simulink model "uncontrolled_group24"  (R2023b)
settings: Solver=ode5  StartTime=0.0  StopTime=333  FixedStep=0.1  RelTol=1e-3
values from neighbouring files (symbols this model uses):
  a = 6939    [Air_Drag_script.m]    (also in main.m = 6939.063; main_group24.m = 6939.063)
  A0 = eye(3)    [Air_Drag_script.m]    (also in main_group24.m)
  ARW = 0.15    [main_group24.m]
  c = 2.99792*10^8    (= 299792000)    [main.m]    (also in main_group24.m)
  e = 0    [Air_Drag_script.m]    (also in main.m = 0.001304; main_group24.m)
  G = [gn, gm, gvali, gsvi]    [main.m]    (also in main_group24.m)
  GyroSampleRate = 10    [main_group24.m]
  H = [hn, hm, hvali, hsvi]    [main.m]    (also in main_group24.m)
  i = deg2rad(97.5307)    [Air_Drag_script.m]    (also in main.m; main_group24.m)
  I_tot = [Ix 0 0; 0 Iy 0; 0 0 Iz]    [data_mass.m]    (also in main_group24.m)
  invI_tot = inv(I_tot)    [data_mass.m]    (also in main_group24.m)
  Ix = J(1,1)    [Air_Drag_script.m]    (also in data_mass.m = 0.0755003333333; main.m = 0.057749855; main_group24.m = 0.0755003333333)
  Iy = J(2,2)    [Air_Drag_script.m]    (also in data_mass.m = 0.0755003333333; main.m = 0.04143542; main_group24.m = 0.0755003333333)
  Iz = J(3,3)    [Air_Drag_script.m]    (also in data_mass.m = 0.055; main.m = 0.024624309; main_group24.m = 0.055)
  m = [0.1; 0.1; 0.1]    [main.m]    (also in main_group24.m)
  MB = [4; 0.1; 0.1; 0.3]    [main.m]    (also in main_group24.m)
  MMnoise = 15e-9*[1; 1; 1]    [main_group24.m]
  MMSampleRate = 1    [main_group24.m]
  mu = 3.98600433e+5    (= 398600.433)    [main.m]    (also in main_group24.m)
  n = 0.0011    [Air_Drag_script.m]    (also in main.m = sqrt(mu/a^3); main_group24.m = sqrt(mu/a^3))
  q0 = [ 1 1 1 1 ]'    [Air_Drag_script.m]    (also in main_group24.m = [0 0 0 1]')
  R_e = 6378    [main.m]    (also in main_group24.m)
  rho_air = 1.65e-13    [Air_Drag_script.m]
  rho_d_MB = 0.1    [main.m]    (also in main_group24.m)
  rho_d_SP = 0.1    [main.m]    (also in main_group24.m)
  rho_s_MB = 0.5    [main.m]    (also in main_group24.m)
  rho_s_SP = 0.1    [main.m]    (also in main_group24.m)
  RRW = 0.3    [main_group24.m]
  SP = [1; 0.3; 0.1; 0.01]    [main.m]    (also in main_group24.m = [0.25; 0.1; 0.3; 0.01])
  w0 = [0 0 0]'    [Air_Drag_script.m]    (also in main.m = [wx0; wy0; wz0]; main_group24.m = [wx0; wy0; wz0])
undefined symbols (not defined in the file or in its folder): Cd, H_0, n_E, P, pan1, pan2, rho_d_body, rho_d_sp, rho_s_body, rho_s_sp, s1, s2, s3, s4, s5, s6, v_rel
libraries: vrlib x40, simulink_extras x13, matrix_library x8, sharedutil x3, simulink x1
(part 2 of 4)

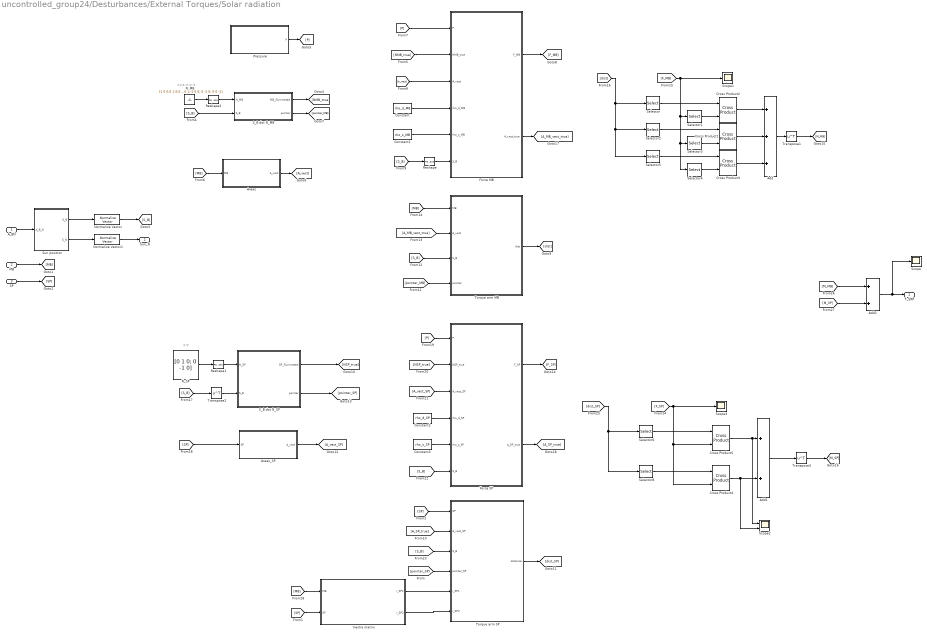
== system uncontrolled_group24/Desturbances/External Torques/Solar radiation ==
  note: x,y,z,-x,-y,-z
  note: y,-y
  A_BN : Inport
  MB : Inport  Port=2
  SP : Inport  Port=3
  Add : Sum  Inputs=3
  Add1 : Sum
  Add2 : Sum
  Areas : Subsystem
  Areas_SP : Subsystem
  Constant : Constant  Value=rho_d_MB
  Constant1 : Constant  Value=rho_s_MB
  Constant2 : Constant  Value=rho_d_SP
  Constant3 : Constant  Value=rho_s_SP
  Cross Product{1..5} (5 alike) : matrix_library/Cross Product
  Force MB : Subsystem
  Force SP : Subsystem
  Inertia matrix : Subsystem
  N_MB : Constant  Value=[1 0 0;0 1 0;0 0 1;-1 0 0; 0 -1 0; 0 0 -1]  VectorParams1D=off
  N_SP : Constant  Value=[0 1 0; 0 -1 0]  VectorParams1D=off
  Normalize Vector : vrlib/Utilities/Normalize Vector  maxzero=0
  Normalize Vector1 : vrlib/Utilities/Normalize Vector  maxzero=0
  Pressure : Subsystem
  Reshape : Reshape  OutputDimensionality=Column vector (2-D)
  Reshape1 : Reshape  OutputDimensionality=Customize  OutputDimensions=[2,3]
  Reshape2 : Reshape  OutputDimensionality=Customize  OutputDimensions=[6,3]
  S_B dot N_MB : Subsystem
  S_B dot N_SP : Subsystem
  Scope : Scope
  Scope1 : Scope
  Scope2 : Scope  NumInputPorts=2
  Scope3 : Scope
  Selector : Selector  NumberOfDimensions=2  InputPortWidth=3  IndexOptions=Index vector (dialog),Index vector (dialog)  Indices=1,[1 2 3]  OutputSizes=1,1
  Selector1 : Selector  NumberOfDimensions=2  InputPortWidth=3  IndexOptions=Index vector (dialog),Index vector (dialog)  Indices=1,[1 2 3]  OutputSizes=1,1
  Selector2 : Selector  NumberOfDimensions=2  InputPortWidth=3  IndexOptions=Index vector (dialog),Index vector (dialog)  Indices=2,[1 2 3]  OutputSizes=1,1
  Selector3 : Selector  NumberOfDimensions=2  InputPortWidth=3  IndexOptions=Index vector (dialog),Index vector (dialog)  Indices=2,[1 2 3]  OutputSizes=1,1
  Selector4 : Selector  NumberOfDimensions=2  InputPortWidth=3  IndexOptions=Index vector (dialog),Index vector (dialog)  Indices=3,[1 2 3]  OutputSizes=1,1
  Selector5 : Selector  NumberOfDimensions=2  InputPortWidth=3  IndexOptions=Index vector (dialog),Index vector (dialog)  Indices=3,[1 2 3]  OutputSizes=1,1
  Selector6 : Selector  NumberOfDimensions=2  InputPortWidth=3  IndexOptions=Index vector (dialog),Index vector (dialog)  Indices=1,[1 2 3]  OutputSizes=1,1
  Selector8 : Selector  NumberOfDimensions=2  InputPortWidth=3  IndexOptions=Index vector (dialog),Index vector (dialog)  Indices=2,[1 2 3]  OutputSizes=1,1
  Sun position : Subsystem
  Torque arm MB : Subsystem
  Torque arm SP : Subsystem
  Transpose1 : Math  Operator=transpose
  Transpose2 : Math  Operator=transpose
  Transpose3 : Math  Operator=transpose
  T_SRP : Outport
  Sun_N : Outport  Port=2
  wires:
  Sun position/1(S_B) -> Normalize Vector/1
  MB/1 -> [MB]
  N_MB/1 -> Reshape2/1
  [NMB_true] -> Force MB/2(NMB_true)
  S_B dot N_MB/1(MB_illuminated) -> [NMB_true]
  [MB] -> Areas/1(MB)
  [S_B] -> S_B dot N_MB/2(S_B)
  [P] -> Force MB/1(P)
  Areas/1(A_vect) -> [A_vect]
  Transpose1/1 -> [M_MB]
  Areas_SP/1(A_vect) -> [A_vect_SP]
  Reshape1/1 -> S_B dot N_SP/1(N_SP)
  Transpose3/1 -> [M_SP]
  Selector2/1 -> Cross Product1/1
  [MB] -> Torque arm MB/1(MB)
  Constant3/1 -> Force SP/5(rho_s_SP)
  [F_SP] -> Cross Product5/2, Cross Product4/2, Scope3/1
  [M_MB] -> Add2/1
  [dist_SP] -> Selector6/1, Selector8/1
  [pointer_SP] -> Torque arm SP/4(pointer_SP)
  Cross Product4/1 -> Scope2/2, Add1/2
  [F_MB] -> Scope1/1, Selector4/1, Selector3/1, Selector1/1
  A_BN/1 -> Sun position/1(A_B_N)
  Add1/1 -> Transpose3/1
  Transpose2/1 -> S_B dot N_SP/2(S_B)
  [SP] -> Areas_SP/1(SP)
  [A_SP_true] -> Torque arm SP/2(A_vect_SP)
  Add/1 -> Transpose1/1
  Torque arm SP/1(distance) -> [dist_SP]
  Reshape2/1 -> S_B dot N_MB/1(N_MB)
  Torque arm MB/1(dist) -> [dist]
  S_B dot N_SP/2(pointer) -> [pointer_SP]
  Force MB/1(F_MB) -> [F_MB]
  Selector/1 -> Cross Product2/1
  [S_B] -> Reshape/1
  [P] -> Force SP/1(P)
  [A_vect] -> Force MB/3(A_vect)
  Selector1/1 -> Cross Product2/2
  Constant1/1 -> Force MB/5(rho_s_MB)
  [A_MB_vect_true] -> Torque arm MB/2(A_vect)
  Pressure/1(P) -> [P]
  Normalize Vector/1 -> [S_B]
  Constant2/1 -> Force SP/4(rho_d_SP)
  Constant/1 -> Force MB/4(rho_d_MB)
  Selector8/1 -> Cross Product4/1
  [dist] -> Selector2/1, Selector5/1, Selector/1
  [NSP_true] -> Force SP/2(NSP_true)
  N_SP/1 -> Reshape1/1
  [S_B] -> Torque arm MB/3(S_B)
  Force SP/2(A_SP_true) -> [A_SP_true]
  [S_B] -> Torque arm SP/3(S_B)
  SP/1 -> [SP]
  Selector4/1 -> Cross Product3/2
  S_B dot N_MB/2(pointer) -> [pointer_MB]
  Force MB/2(A_vect_true) -> [A_MB_vect_true]
  [pointer_MB] -> Torque arm MB/4(pointer)
  Add2/1 -> Scope/1, T_SRP/1
  Selector3/1 -> Cross Product1/2
  [S_B] -> Force SP/6(S_B)
  [S_B] -> Transpose2/1
  Cross Product5/1 -> Scope2/1, Add1/1
  [A_vect_SP] -> Force SP/3(A_vect_SP)
  Reshape/1 -> Force MB/6(S_B)
  Cross Product2/1 -> Add/1
  Force SP/1(F_SP) -> [F_SP]
  S_B dot N_SP/1(SP_illuminated) -> [NSP_true]
  Selector6/1 -> Cross Product5/1
  Selector5/1 -> Cross Product3/1
  Cross Product1/1 -> Add/2
  [M_SP] -> Add2/2
  [SP] -> Torque arm SP/1(SP)
  Cross Product3/1 -> Add/3
  [SP] -> Inertia matrix/2(SP)
  [MB] -> Inertia matrix/1(MB)
  Inertia matrix/1(r_SP1) -> Torque arm SP/5(r_SP1)
  Inertia matrix/2(r_SP2) -> Torque arm SP/6(r_SP2)
  Sun position/2(S_N) -> Normalize Vector1/1
  Normalize Vector1/1 -> Sun_N/1

== system uncontrolled_group24/Desturbances/Orbital Mechanics/Sat Position magnitude ==
  note: 1+e cos(theta)
  note: a(1-e^2)
  note: Denominator
  note: Numerator
  theta : Inport
  Constant : Constant  Value=a
  Constant1 : Constant
  Constant3 : Constant  Value=e
  Constant4 : Constant
  Constant5 : Constant  Value=e
  Cos : Trigonometry  Operator=cos
  Divide : Product  Inputs=*/
  Product : Product
  Product1 : Product
  Square1 : Math  Operator=square
  Sum : Sum
  Sum1 : Sum  Inputs=+-
  r : Outport
  wires:
  Product1/1 -> Sum/1
  Sum1/1 -> Product/2
  Constant1/1 -> Sum1/1
  Sum/1 -> Divide/2
  Square1/1 -> Sum1/2
  Constant3/1 -> Product1/2
  Constant4/1 -> Sum/2
  Constant/1 -> Product/1
  Constant5/1 -> Square1/1
  Cos/1 -> Product1/1
  Product/1 -> Divide/1
  theta/1 -> Cos/1
  Divide/1 -> r/1

== system uncontrolled_group24/Desturbances/Orbital Mechanics/Sat True Anomaly ==
  note: (1-e^2)^3/2
  note: n ( 1+e cos(theta))^2
  note: Denominator
  note: Numerator
  Constant : Constant  Value=n
  Constant1 : Constant
  Constant2 : Constant  Value=e
  Constant3 : Constant
  Constant4 : Constant  Value=e
  Constant5 : Constant  Value=3/2
  Cos : Trigonometry  Operator=cos
  Divide : Product  Inputs=*/
  Integrator : Integrator
  Power : Math  Operator=pow
  Product : Product
  Product1 : Product
  Square : Math  Operator=square
  Square1 : Math  Operator=square
  Sum : Sum
  Sum1 : Sum  Inputs=|+-
  theta : Outport
  wires:
  Sum/1 -> Square/1
  Integrator/1 -> theta/1, Cos/1  "theta"
  Square/1 -> Product1/2
  Constant5/1 -> Power/2
  Constant3/1 -> Sum1/1
  Product1/1 -> Divide/1
  Constant/1 -> Product1/1
  Divide/1 -> Integrator/1  "theta_dot"
  Square1/1 -> Sum1/2
  Product/1 -> Sum/2
  Power/1 -> Divide/2
  Constant1/1 -> Sum/1
  Constant2/1 -> Product/1
  Constant4/1 -> Square1/1
  Cos/1 -> Product/2
  Sum1/1 -> Power/1

== system uncontrolled_group24/Desturbances/Orbital Mechanics/Sat position vector in inertial frame ==
  note: r_N = r [cos(theta)
      | 		sin(theta)cos(i)
      | 		sin(theta)sin(i)]
  r : Inport
  theta : Inport  Port=2
  Cos : Trigonometry  Operator=cos
  Cos1 : Trigonometry  Operator=cos
  Orbit Inclination : Constant  Value=i
  Product : Product
  Product1 : Product
  Product2 : Product
  Sin : Trigonometry
  Sin1 : Trigonometry
  Vector Concatenate : Concatenate  NumInputs=3  Mode=Multidimensional array
  r_N : Outport
  wires:
  Sin/1 -> Product1/1, Product/1
  Product/1 -> Vector Concatenate/2
  Sin1/1 -> Product1/2
  r/1 -> Product2/1
  Orbit Inclination/1 -> Sin1/1, Cos1/1
  Vector Concatenate/1 -> Product2/2
  theta/1 -> Cos/1, Sin/1
  Cos/1 -> Vector Concatenate/1
  Cos1/1 -> Product/2
  Product1/1 -> Vector Concatenate/3
  Product2/1 -> r_N/1

== system uncontrolled_group24/Desturbances/Relative Attitude/A_BL ==
  A_BN : Inport
  A_LN : Inport  Port=2
  Matrix Multiply : Product  Multiplication=Matrix(*)
  To Workspace : ToWorkspace  VariableName=A_BL  SampleTime=-1
  Transpose1 : matrix_library/Transpose
  A_BL : Outport
  wires:
  A_BN/1 -> Matrix Multiply/1
  A_LN/1 -> Transpose1/1
  Transpose1/1 -> Matrix Multiply/2
  Matrix Multiply/1 -> A_BL/1, To Workspace/1

== system uncontrolled_group24/Desturbances/Relative Attitude/A_LN ==
  theta : Inport
  Constant : Constant  Value=0
  Constant1 : Constant  Value=[0; 0; 1]
  Constant2 : Constant  Value=[1 0 0; 0 cos(i) sin(i); 0 -sin(i) cos(i)]
  Cos : Trigonometry  Operator=cos
  Gain : Gain  Gain=[1; -1; 1]
  Matrix Concatenate : Concatenate  NumInputs=3  Mode=Multidimensional array  ConcatenateDimension=2
  Product : Product  Multiplication=Matrix(*)
  Selector : Selector  InputPortWidth=3  IndexOptions=Index vector (dialog)  Indices=[3 2 1]  OutputSizes=1
  Selector1 : Selector  InputPortWidth=3  IndexOptions=Index vector (dialog)  Indices=[2 3 1]  OutputSizes=1
  Sin : Trigonometry
  To Workspace : ToWorkspace  VariableName=A_LN  SampleTime=-1
  Vector Concatenate : Concatenate  NumInputs=3
  A_LN : Outport
  wires:
  Matrix Concatenate/1 -> Product/1
  theta/1 -> Sin/1, Cos/1
  Gain/1 -> Matrix Concatenate/1
  Vector Concatenate/1 -> Selector1/1, Selector/1
  Sin/1 -> Vector Concatenate/3
  Selector/1 -> Matrix Concatenate/2
  Selector1/1 -> Gain/1
  Product/1 -> A_LN/1, To Workspace/1
  Constant1/1 -> Matrix Concatenate/3
  Cos/1 -> Vector Concatenate/2
  Constant/1 -> Vector Concatenate/1
  Constant2/1 -> Product/2

== system uncontrolled_group24/Sensors/Magnetometer/Subsystem ==
  Constant : Constant
  Display : Display
  Gain : Gain  Gain=[1; -1; 1]
  Gain1 : Gain  Gain=[1; 1; -1]
  Gain2 : Gain  Gain=[-1; 1; 1]
  Matrix Concatenate : Concatenate  NumInputs=3  Mode=Multidimensional array  ConcatenateDimension=2
  Random Number : RandomNumber  Variance=deg2rad(0.1)^2  Seed=5  SampleTime=1/MMSampleRate
  Random Number1 : RandomNumber  Variance=deg2rad(0.1)^2  Seed=6  SampleTime=1/MMSampleRate
  Random Number2 : RandomNumber  Variance=deg2rad(0.1)^2  Seed=7  SampleTime=1/MMSampleRate
  Selector : Selector  InputPortWidth=4  IndexOptions=Index vector (dialog)  Indices=[1 4 3]  OutputSizes=1
  Selector1 : Selector  InputPortWidth=4  IndexOptions=Index vector (dialog)  Indices=[4 1 2]  OutputSizes=1
  Selector2 : Selector  InputPortWidth=4  IndexOptions=Index vector (dialog)  Indices=[3 2 1]  OutputSizes=1
  Vector Concatenate : Concatenate  NumInputs=4
  A_epsMM : Outport
  wires:
  Selector2/1 -> Gain2/1
  Selector/1 -> Gain/1
  Gain/1 -> Matrix Concatenate/1
  Random Number/1 -> Vector Concatenate/2
  Matrix Concatenate/1 -> Display/1, A_epsMM/1
  Selector1/1 -> Gain1/1
  Vector Concatenate/1 -> Selector2/1, Selector/1, Selector1/1
  Gain2/1 -> Matrix Concatenate/3
  Constant/1 -> Vector Concatenate/1
  Gain1/1 -> Matrix Concatenate/2
  Random Number2/1 -> Vector Concatenate/4
  Random Number1/1 -> Vector Concatenate/3

== system uncontrolled_group24/Sensors/Sun Sensor/Subsystem ==
  note: A31
  note: A33
  note: A32
  note: A23
  note: A22
  note: A21
  note: A13
  note: A12
  note: A11
  Cos : Trigonometry  Operator=cos
  Cos1 : Trigonometry  Operator=cos
  Cos2 : Trigonometry  Operator=cos
  Create 3x3 Matrix : sharedutil/Create 3x3 Matrix  aMode=aMode
  Gain1 : Gain  Gain=-1
  Gain3 : Gain  Gain=-1
  Gain4 : Gain
  Product{,1,3,5..6,8,10..11} (8 alike) : Product
  Product{2,4,7,9} (4 alike) : Product  Inputs=3
  Sin : Trigonometry
  Sin1 : Trigonometry
  Sin2 : Trigonometry
  Sum : Sum
  Sum1 : Sum  Inputs=-+
  Sum2 : Sum  Inputs=-+
  Sum3 : Sum
  phi : RandomNumber  Variance=(1/8*pi/180)^2  Seed=2  SampleTime=0.2
  psi : RandomNumber  Variance=(1/8*pi/180)^2  SampleTime=0.2
  th : RandomNumber  Variance=(1/8*pi/180)^2  Seed=1  SampleTime=0.2
  A_eps : Outport
  wires:
  psi/1 -> Cos/1, Sin/1
  th/1 -> Sin1/1, Cos1/1
  phi/1 -> Sin2/1, Cos2/1
  Product2/1 -> Sum/1
  Product1/1 -> Sum/2
  Product3/1 -> Sum1/2
  Product4/1 -> Sum1/1
  Product7/1 -> Sum2/1
  Product6/1 -> Sum2/2
  Product9/1 -> Sum3/1
  Product8/1 -> Sum3/2
  Gain4/1 -> Create 3x3 Matrix/7  "A31"
  Product/1 -> Create 3x3 Matrix/1  "A11"
  Sum/1 -> Create 3x3 Matrix/2  "A12"
  Sum1/1 -> Create 3x3 Matrix/3  "A13"
  Product5/1 -> Gain1/1
  Sum2/1 -> Create 3x3 Matrix/5  "A22"
  Sum3/1 -> Create 3x3 Matrix/6  "A23"
  Product10/1 -> Gain3/1
  Product11/1 -> Create 3x3 Matrix/9  "A33"
  Gain1/1 -> Create 3x3 Matrix/4  "A21"
  Gain3/1 -> Create 3x3 Matrix/8  "A32"
  Cos/1 -> Product8/1, Product6/1, Product4/1, Product2/1, Product/1  "cos(psi)"
  Cos1/1 -> Product/2, Product11/1, Product10/1, Product5/2  "cos(th)"
  Sin1/1 -> Gain4/1, Product9/2, Product7/2, Product2/2, Product4/2  "sin(th)"
  Sin2/1 -> Product7/3, Product3/2, Product2/3, Product8/2, Product10/2  "sin(phi)"
  Sin/1 -> Product3/1, Product5/1, Product7/1, Product9/1, Product1/1  "sin(psi)"
  Cos2/1 -> Product6/2, Product4/3, Product1/2, Product9/3, Product11/2  "cos(phi)"
  Create 3x3 Matrix/1 -> A_eps/1  "A_eps"

== system uncontrolled_group24/errormeasure/IJK_error/I_Error ==
  A_BN_estimated : Inport
  I : Inport  Port=2
  A_B_N_ea : Inport  Port=3
  Acos : Trigonometry  Operator=acos
  Dot Product : DotProduct  OutDataTypeStr=Inherit: Inherit via internal rule
  MatrixMultiply : Product  Multiplication=Matrix(*)
  MatrixMultiply1 : Product  Multiplication=Matrix(*)
  Normalize Vector : vrlib/Utilities/Normalize Vector  maxzero=0
  Normalize Vector1 : vrlib/Utilities/Normalize Vector  maxzero=0
  Radians to Degrees : simulink_extras/Transformations/Radians to Degrees
  Degrees out : Outport
  wires:
  MatrixMultiply1/1 -> Normalize Vector/1
  Dot Product/1 -> Acos/1
  I/1 -> MatrixMultiply1/2, MatrixMultiply/2
  Normalize Vector1/1 -> Dot Product/2
  Normalize Vector/1 -> Dot Product/1
  Acos/1 -> Radians to Degrees/1  "Theta_err"
  A_BN_estimated/1 -> MatrixMultiply1/1
  MatrixMultiply/1 -> Normalize Vector1/1
  A_B_N_ea/1 -> MatrixMultiply/1
  Radians to Degrees/1 -> Degrees out/1

== system uncontrolled_group24/errormeasure/IJK_error/J_Error ==
  A_BN_estimated : Inport
  J : Inport  Port=2
  A_B_N_ea : Inport  Port=3
  Acos : Trigonometry  Operator=acos
  Dot Product : DotProduct  OutDataTypeStr=Inherit: Inherit via internal rule
  MatrixMultiply : Product  Multiplication=Matrix(*)
  MatrixMultiply1 : Product  Multiplication=Matrix(*)
  Normalize Vector : vrlib/Utilities/Normalize Vector  maxzero=0
  Normalize Vector1 : vrlib/Utilities/Normalize Vector  maxzero=0
  Radians to Degrees : simulink_extras/Transformations/Radians to Degrees
  Degrees out : Outport
  wires:
  MatrixMultiply1/1 -> Normalize Vector/1
  Dot Product/1 -> Acos/1
  J/1 -> MatrixMultiply1/2, MatrixMultiply/2
  Normalize Vector1/1 -> Dot Product/2
  Normalize Vector/1 -> Dot Product/1
  Acos/1 -> Radians to Degrees/1  "Theta_err"
  A_BN_estimated/1 -> MatrixMultiply1/1
  MatrixMultiply/1 -> Normalize Vector1/1
  A_B_N_ea/1 -> MatrixMultiply/1
  Radians to Degrees/1 -> Degrees out/1

== system uncontrolled_group24/errormeasure/IJK_error/K_Error ==
  A_BN_estimated : Inport
  K : Inport  Port=2
  A_B_N_ea : Inport  Port=3
  Acos : Trigonometry  Operator=acos
  Dot Product : DotProduct  OutDataTypeStr=Inherit: Inherit via internal rule
  MatrixMultiply : Product  Multiplication=Matrix(*)
  MatrixMultiply1 : Product  Multiplication=Matrix(*)
  Normalize Vector : vrlib/Utilities/Normalize Vector  maxzero=0
  Normalize Vector1 : vrlib/Utilities/Normalize Vector  maxzero=0
  Radians to Degrees : simulink_extras/Transformations/Radians to Degrees
  Degrees out : Outport
  wires:
  MatrixMultiply1/1 -> Normalize Vector/1
  Dot Product/1 -> Acos/1
  K/1 -> MatrixMultiply1/2, MatrixMultiply/2
  Normalize Vector1/1 -> Dot Product/2
  Normalize Vector/1 -> Dot Product/1
  Acos/1 -> Radians to Degrees/1  "Theta_err"
  A_BN_estimated/1 -> MatrixMultiply1/1
  MatrixMultiply/1 -> Normalize Vector1/1
  A_B_N_ea/1 -> MatrixMultiply/1
  Radians to Degrees/1 -> Degrees out/1

== system uncontrolled_group24/Desturbances/External Torques/M_GG/GG Torque1 ==
  c1 : Inport
  c2 : Inport  Port=2
  c3 : Inport  Port=3
  r : Inport  Port=4
  Constant5 : Constant  Value=3
  Constant6 : Constant  Value=3*mu
  Divide3 : Product  Inputs=*/
  Gain1 : Gain  Gain=Iz-Iy
  Gain2 : Gain  Gain=Ix-Iz
  Gain3 : Gain  Gain=Iy-Ix
  Mux1 : Mux  Inputs=3
  Pow1 : Math  Operator=pow  RndMeth=Zero
  Product{1..2,6..9} (6 alike) : Product
  M_GG : Outport
  wires:
  Gain1/1 -> Mux1/1
  Product7/1 -> Gain1/1
  Gain3/1 -> Mux1/3
  Product2/1 -> Product8/1
  r/1 -> Pow1/1
  Product6/1 -> Product9/1
  Product1/1 -> Product7/1
  Constant6/1 -> Divide3/1
  Product8/1 -> Gain2/1
  Pow1/1 -> Divide3/2
  c2/1 -> Product6/2, Product1/1
  Mux1/1 -> M_GG/1
  Product9/1 -> Gain3/1
  Constant5/1 -> Pow1/2
  Gain2/1 -> Mux1/2
  c3/1 -> Product1/2, Product2/2
  c1/1 -> Product6/1, Product2/1
  Divide3/1 -> Product7/2, Product8/2, Product9/2

== system uncontrolled_group24/Desturbances/External Torques/M_GG/c1, c2, c3 ==
  A_BL : Inport
  Constant1 : Constant  Value=[1; 0; 0]
  Demux : Demux  Outputs=3
  Product1 : Product  Multiplication=Matrix(*)
  c1 : Outport
  c2 : Outport  Port=2
  c3 : Outport  Port=3
  wires:
  Demux/2 -> c2/1
  Product1/1 -> Demux/1
  Demux/1 -> c1/1
  Demux/3 -> c3/1
  Constant1/1 -> Product1/2
  A_BL/1 -> Product1/1

== system uncontrolled_group24/Desturbances/External Torques/SRP con frecce/SRP ==
  r_s_B : Inport
  Subsystem : Subsystem
  Subsystem1 : Subsystem
  Subsystem2 : Subsystem
  Subsystem3 : Subsystem
  Subsystem4 : Subsystem
  Subsystem5 : Subsystem
  Subsystem6 : Subsystem
  Subsystem7 : Subsystem
  Subsystem8 : Subsystem
  Subsystem9 : Subsystem
  Sum : Sum  Inputs=++++++++++
  Tsrp : Outport
  wires:
  r_s_B/1 -> Subsystem2/1(r_s_B), Subsystem/1(r_s_B), Subsystem1/1(r_s_B), Subsystem4/1(r_s_B), Subsystem3/1(r_s_B), Subsystem7/1(r_s_B), Subsystem5/1(r_s_B), Subsystem6/1(r_s_B), Subsystem9/1(r_s_B), Subsystem8/1(r_s_B)
  Subsystem2/1(pan1) -> Sum/1
  Subsystem/1(pan2) -> Sum/2
  Subsystem1/1(pan3) -> Sum/3
  Subsystem4/1(pan4) -> Sum/4
  Subsystem3/1(pan5) -> Sum/5
  Subsystem7/1(pan6) -> Sum/6
  Subsystem5/1(ps1) -> Sum/7
  Subsystem6/1(ps2) -> Sum/8
  Subsystem9/1(ps3) -> Sum/9
  Subsystem8/1(ps4) -> Sum/10
  Sum/1 -> Tsrp/1

== system uncontrolled_group24/Desturbances/External Torques/Solar radiation/Areas ==
  MB : Inport
  Demux : Demux
  Mux : Mux  Inputs=3
  Product1 : Product
  Product2 : Product
  Product4 : Product
  Reshape : Reshape  OutputDimensionality=Column vector (2-D)
  Terminator : Terminator
  A_vect : Outport
  wires:
  Product2/1 -> Mux/2  "a*h"
  Product4/1 -> Mux/1  "b*h"
  MB/1 -> Demux/1
  Product1/1 -> Mux/3  "a*b"
  Demux/1 -> Terminator/1
  Demux/2 -> [a]
  Demux/3 -> [b]
  Demux/4 -> [h]
  [b] -> Product4/1
  [h] -> Product4/2
  [h] -> Product2/2
  [b] -> Product1/2
  [a] -> Product2/1
  [a] -> Product1/1
  Mux/1 -> Reshape/1
  Reshape/1 -> A_vect/1

== system uncontrolled_group24/Desturbances/External Torques/Solar radiation/Areas_SP ==
  SP : Inport
  Demux : Demux
  Product1 : Product
  Terminator : Terminator
  Terminator1 : Terminator
  A_vect : Outport
  wires:
  [a] -> Product1/1
  [b] -> Product1/2
  Demux/4 -> Terminator1/1
  Demux/3 -> [b]
  Demux/2 -> [a]
  Demux/1 -> Terminator/1
  Product1/1 -> A_vect/1  "a*b"
  SP/1 -> Demux/1

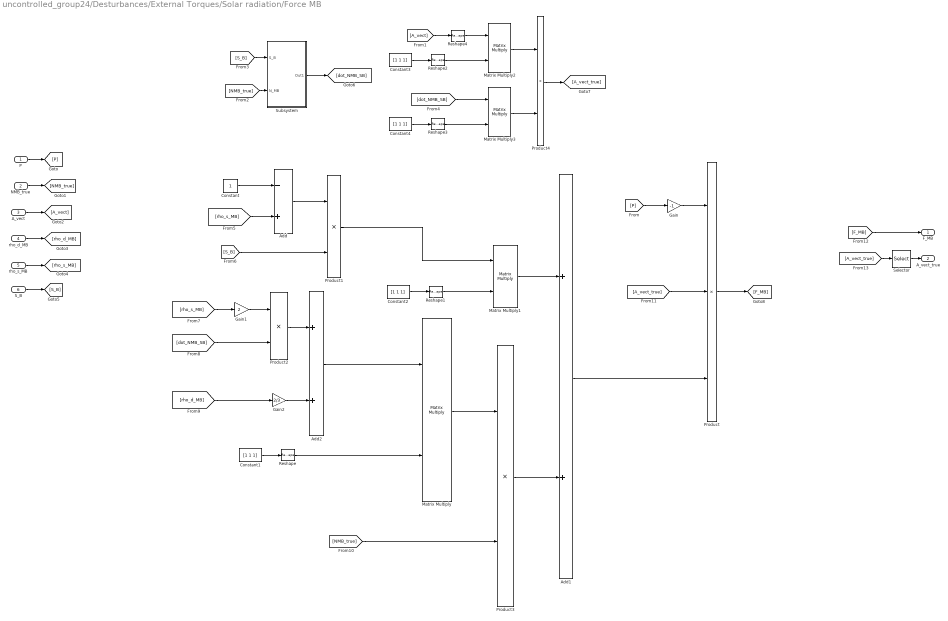
== system uncontrolled_group24/Desturbances/External Torques/Solar radiation/Force MB ==
  P : Inport
  NMB_true : Inport  Port=2
  A_vect : Inport  Port=3
  rho_d_MB : Inport  Port=4
  rho_s_MB : Inport  Port=5
  S_B : Inport  Port=6
  Add : Sum  Inputs=-+
  Add1 : Sum
  Add2 : Sum
  Constant : Constant
  Constant{1..4} (4 alike) : Constant  Value=[1 1 1]
  Gain : Gain  Gain=-1
  Gain1 : Gain  Gain=2
  Gain2 : Gain  Gain=2/3
  Matrix Multiply{,1..3} (4 alike) : Product  Multiplication=Matrix(*)
  Product : Product  Inputs=3
  Product{1..4} (4 alike) : Product
  Reshape{,1..3} (4 alike) : Reshape  OutputDimensionality=Row vector (2-D)
  Reshape4 : Reshape  OutputDimensionality=Column vector (2-D)
  Selector : Selector  NumberOfDimensions=2  InputPortWidth=3  IndexOptions=Index vector (dialog),Index vector (dialog)  Indices=[1 2 3],1  OutputSizes=1,1
  Subsystem : Subsystem
  F_MB : Outport
  A_vect_true : Outport  Port=2
  wires:
  P/1 -> [P]
  NMB_true/1 -> [NMB_true]
  A_vect/1 -> [A_vect]
  rho_d_MB/1 -> [rho_d_MB]
  rho_s_MB/1 -> [rho_s_MB]
  S_B/1 -> [S_B]
  [P] -> Gain/1
  Gain/1 -> Product/1
  [NMB_true] -> Subsystem/2(N_MB)
  [S_B] -> Subsystem/1(S_B)
  Subsystem/1(Out1) -> [dot_NMB_SB]
  [rho_s_MB] -> Add/2
  Constant/1 -> Add/1
  Add/1 -> Product1/1
  [S_B] -> Product1/2
  [rho_s_MB] -> Gain1/1
  [dot_NMB_SB] -> Product2/2
  Gain1/1 -> Product2/1
  Product2/1 -> Add2/1
  Gain2/1 -> Add2/2
  [rho_d_MB] -> Gain2/1
  [NMB_true] -> Product3/2
  Product3/1 -> Add1/2
  Add1/1 -> Product/3
  Constant1/1 -> Reshape/1
  Matrix Multiply/1 -> Product3/1
  Add2/1 -> Matrix Multiply/1
  Reshape/1 -> Matrix Multiply/2
  Matrix Multiply1/1 -> Add1/1
  Product1/1 -> Matrix Multiply1/1
  Constant2/1 -> Reshape1/1
  Reshape1/1 -> Matrix Multiply1/2
  Reshape2/1 -> Matrix Multiply2/2
  Constant3/1 -> Reshape2/1
  Reshape3/1 -> Matrix Multiply3/2
  Constant4/1 -> Reshape3/1
  [A_vect] -> Reshape4/1
  Reshape4/1 -> Matrix Multiply2/1
  [dot_NMB_SB] -> Matrix Multiply3/1
  Matrix Multiply2/1 -> Product4/1
  Matrix Multiply3/1 -> Product4/2
  Product4/1 -> [A_vect_true]
  [A_vect_true] -> Product/2
  Product/1 -> [F_MB]
  [F_MB] -> F_MB/1
  [A_vect_true] -> Selector/1
  Selector/1 -> A_vect_true/1

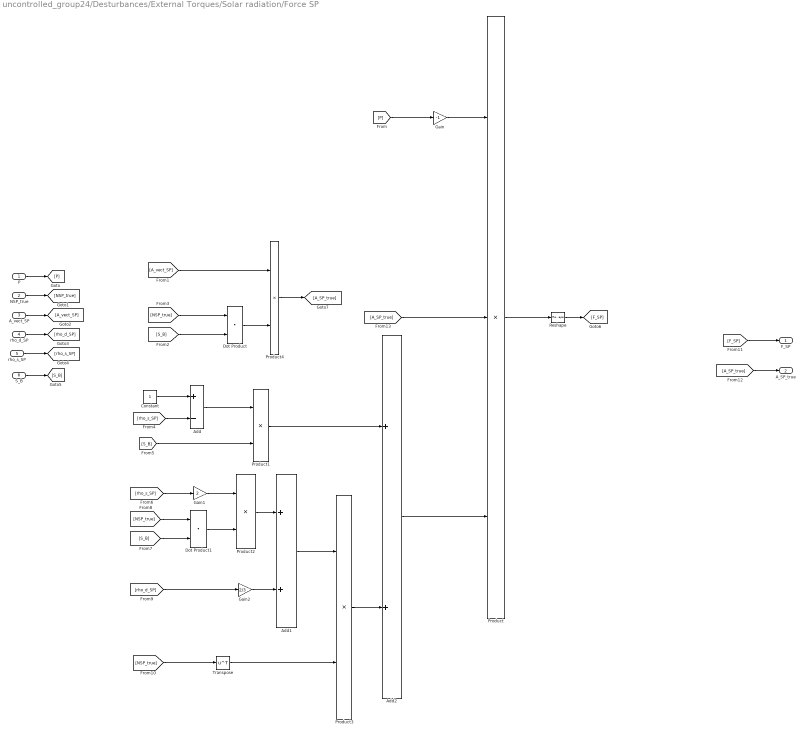
== system uncontrolled_group24/Desturbances/External Torques/Solar radiation/Force SP ==
  P : Inport
  NSP_true : Inport  Port=2
  A_vect_SP : Inport  Port=3
  rho_d_SP : Inport  Port=4
  rho_s_SP : Inport  Port=5
  S_B : Inport  Port=6
  Add : Sum  Inputs=+-
  Add1 : Sum
  Add2 : Sum
  Constant : Constant
  Dot Product : DotProduct  OutDataTypeStr=Inherit: Inherit via internal rule
  Dot Product1 : DotProduct  OutDataTypeStr=Inherit: Inherit via internal rule
  Gain : Gain  Gain=-1
  Gain1 : Gain  Gain=2
  Gain2 : Gain  Gain=2/3
  Product : Product  Inputs=3
  Product{1..4} (4 alike) : Product
  Reshape : Reshape  OutputDimensionality=Row vector (2-D)
  Transpose : Math  Operator=transpose
  F_SP : Outport
  A_SP_true : Outport  Port=2
  wires:
  P/1 -> [P]
  NSP_true/1 -> [NSP_true]
  A_vect_SP/1 -> [A_vect_SP]
  rho_d_SP/1 -> [rho_d_SP]
  rho_s_SP/1 -> [rho_s_SP]
  S_B/1 -> [S_B]
  Product/1 -> Reshape/1
  [P] -> Gain/1
  Gain/1 -> Product/1
  [S_B] -> Dot Product/2
  [NSP_true] -> Dot Product/1
  Constant/1 -> Add/1
  [rho_s_SP] -> Add/2
  Add/1 -> Product1/1
  [S_B] -> Product1/2
  [rho_s_SP] -> Gain1/1
  [NSP_true] -> Dot Product1/1
  [S_B] -> Dot Product1/2
  Dot Product1/1 -> Product2/2
  Gain1/1 -> Product2/1
  Product2/1 -> Add1/1
  [rho_d_SP] -> Gain2/1
  Gain2/1 -> Add1/2
  [NSP_true] -> Transpose/1
  Add1/1 -> Product3/1
  Product1/1 -> Add2/1
  Product3/1 -> Add2/2
  Transpose/1 -> Product3/2
  Add2/1 -> Product/3
  Reshape/1 -> [F_SP]
  [F_SP] -> F_SP/1
  Dot Product/1 -> Product4/2
  [A_vect_SP] -> Product4/1
  Product4/1 -> [A_SP_true]
  [A_SP_true] -> A_SP_true/1
  [A_SP_true] -> Product/2

== system uncontrolled_group24/Desturbances/External Torques/Solar radiation/Inertia matrix ==
  MB : Inport
  SP : Inport  Port=2
  Demux : Demux
  Demux1 : Demux
  Terminator{,1..5} (6 alike) : Terminator
  r_SP : Subsystem
  r_SP1 : Outport
  r_SP2 : Outport  Port=2
  wires:
  [a_MB] -> r_SP/2(a_MB)
  Demux/1 -> Terminator5/1
  SP/1 -> Demux/1
  Demux1/2 -> [a_MB]
  Demux1/3 -> Terminator/1
  Demux1/1 -> Terminator2/1
  Demux1/4 -> Terminator1/1
  MB/1 -> Demux1/1
  Demux/4 -> Terminator3/1
  Demux/2 -> Terminator4/1
  r_SP/2(r_SP2) -> r_SP2/1
  Demux/3 -> [b_SP]
  [b_SP] -> r_SP/1(b_SP)
  r_SP/1(r_SP1) -> r_SP1/1

== system uncontrolled_group24/Desturbances/External Torques/Solar radiation/Pressure ==
  Constant6 : Constant  Value=1358
  Constant7 : Constant  Value=c
  Product8 : Product
  Reciprocal : Product  Inputs=/
  P : Outport
  wires:
  Constant6/1 -> Product8/1
  Reciprocal/1 -> Product8/2
  Product8/1 -> P/1
  Constant7/1 -> Reciprocal/1

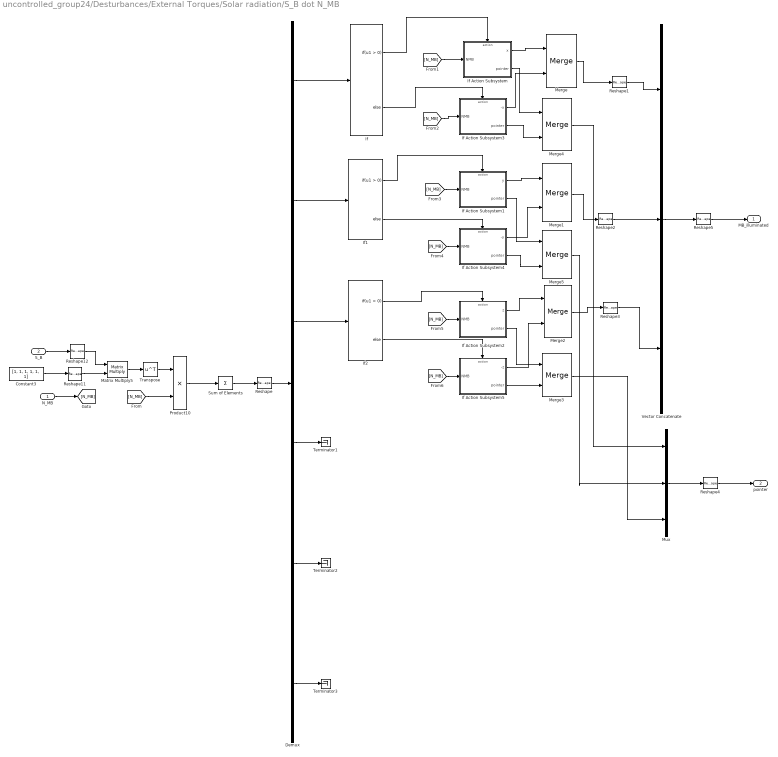
== system uncontrolled_group24/Desturbances/External Torques/Solar radiation/S_B dot N_MB ==
  N_MB : Inport
  S_B : Inport  Port=2
  Constant3 : Constant  Value=[1, 1, 1, 1, 1, 1]  VectorParams1D=off
  Demux : Demux  Outputs=6
  If : If
  If Action Subsystem : Subsystem  TreatAsAtomicUnit=on
  If Action Subsystem1 : Subsystem  TreatAsAtomicUnit=on
  If Action Subsystem2 : Subsystem  TreatAsAtomicUnit=on
  If Action Subsystem3 : Subsystem  TreatAsAtomicUnit=on
  If Action Subsystem4 : Subsystem  TreatAsAtomicUnit=on
  If Action Subsystem5 : Subsystem  TreatAsAtomicUnit=on
  If1 : If
  If2 : If
  Matrix Multiply5 : Product  Multiplication=Matrix(*)
  Merge{,1..5} (6 alike) : Merge
  Mux : Mux  Inputs=3
  Product10 : Product
  Reshape{,1..4,12} (6 alike) : Reshape  OutputDimensionality=Column vector (2-D)
  Reshape11 : Reshape  OutputDimensionality=Row vector (2-D)
  Reshape5 : Reshape  OutputDimensionality=Customize  OutputDimensions=[3,3]
  Sum of Elements : Sum  Inputs=+  CollapseMode=Specified dimension  CollapseDim=2
  Terminator1 : Terminator
  Terminator2 : Terminator
  Terminator3 : Terminator
  Transpose : Math  Operator=transpose
  Vector Concatenate : Concatenate  NumInputs=3
  MB_illuminated : Outport
  pointer : Outport  Port=2
  wires:
  Reshape12/1 -> Matrix Multiply5/1
  Matrix Multiply5/1 -> Transpose/1
  Product10/1 -> Sum of Elements/1
  Reshape11/1 -> Matrix Multiply5/2
  Constant3/1 -> Reshape11/1
  S_B/1 -> Reshape12/1
  Sum of Elements/1 -> Reshape/1
  Reshape/1 -> Demux/1
  Demux/1 -> If/1
  If/1 -> If Action Subsystem/Action
  If/2 -> If Action Subsystem3/Action
  N_MB/1 -> [N_MB]
  [N_MB] -> Product10/2
  [N_MB] -> If Action Subsystem/1(NMB)
  Demux/4 -> Terminator1/1
  Demux/5 -> Terminator2/1
  Demux/6 -> Terminator3/1
  Demux/2 -> If1/1
  If1/1 -> If Action Subsystem1/Action
  [N_MB] -> If Action Subsystem3/1(NMB)
  [N_MB] -> If Action Subsystem1/1(NMB)
  If1/2 -> If Action Subsystem4/Action
  [N_MB] -> If Action Subsystem4/1(NMB)
  If Action Subsystem3/1(-x) -> Merge/2
  If Action Subsystem/1(x) -> Merge/1
  If Action Subsystem1/1(y) -> Merge1/1
  If Action Subsystem2/1(z) -> Merge2/1
  If Action Subsystem5/1(-z) -> Merge2/2
  Demux/3 -> If2/1
  If2/1 -> If Action Subsystem2/Action
  If2/2 -> If Action Subsystem5/Action
  [N_MB] -> If Action Subsystem2/1(NMB)
  [N_MB] -> If Action Subsystem5/1(NMB)
  Merge/1 -> Reshape1/1
  Merge1/1 -> Reshape2/1
  Merge2/1 -> Reshape3/1
  Reshape1/1 -> Vector Concatenate/1
  Reshape2/1 -> Vector Concatenate/2
  Reshape3/1 -> Vector Concatenate/3
  Vector Concatenate/1 -> Reshape5/1
  If Action Subsystem4/1(-y) -> Merge1/2
  If Action Subsystem/2(pointer) -> Merge4/1
  If Action Subsystem3/2(pointer) -> Merge4/2
  If Action Subsystem1/2(pointer) -> Merge5/1
  If Action Subsystem4/2(pointer) -> Merge5/2
  If Action Subsystem2/2(pointer) -> Merge3/1
  If Action Subsystem5/2(pointer) -> Merge3/2
  Merge4/1 -> Mux/1
  Merge5/1 -> Mux/2
  Merge3/1 -> Mux/3
  Mux/1 -> Reshape4/1
  Reshape4/1 -> pointer/1
  Reshape5/1 -> MB_illuminated/1
  Transpose/1 -> Product10/1

== system uncontrolled_group24/Desturbances/External Torques/Solar radiation/S_B dot N_SP ==
  N_SP : Inport
  S_B : Inport  Port=2
  Constant3 : Constant  Value=[1, 1]
  Demux : Demux  Outputs=2
  If : If
  If Action Subsystem : Subsystem  TreatAsAtomicUnit=on
  If Action Subsystem1 : Subsystem  TreatAsAtomicUnit=on
  If1 : If
  Matrix Multiply5 : Product  Multiplication=Matrix(*)
  Merge : Merge
  Merge1 : Merge
  Product10 : Product
  Reshape11 : Reshape  OutputDimensionality=Row vector (2-D)
  Reshape12 : Reshape  OutputDimensionality=Column vector (2-D)
  Sum of Elements : Sum  Inputs=+  CollapseMode=Specified dimension  CollapseDim=2
  Terminator : Terminator
  Terminator1 : Terminator
  Transpose : Math  Operator=transpose
  SP_illuminated : Outport
  pointer : Outport  Port=2
  wires:
  [N_SP] -> Product10/2
  N_SP/1 -> [N_SP]
  Sum of Elements/1 -> Demux/1
  S_B/1 -> Reshape12/1
  Constant3/1 -> Reshape11/1
  Reshape11/1 -> Matrix Multiply5/2
  Product10/1 -> Sum of Elements/1
  Matrix Multiply5/1 -> Transpose/1
  Reshape12/1 -> Matrix Multiply5/1
  Transpose/1 -> Product10/1
  Demux/1 -> If/1
  If/1 -> If Action Subsystem/Action
  Demux/2 -> If1/1
  [N_SP] -> If Action Subsystem/1(N_SP)
  [N_SP] -> If Action Subsystem1/1(N_SP)
  If1/1 -> If Action Subsystem1/Action
  If1/2 -> Terminator/1
  If/2 -> Terminator1/1
  If Action Subsystem/1(true_NSP) -> Merge/1
  If Action Subsystem1/1(true_NSP) -> Merge/2
  If Action Subsystem/2(pointer) -> Merge1/1
  If Action Subsystem1/2(pointer) -> Merge1/2
  Merge/1 -> SP_illuminated/1
  Merge1/1 -> pointer/1

== system uncontrolled_group24/Desturbances/External Torques/Solar radiation/Sun position ==
  A_B_N : Inport
  Clock : Clock
  Constant : Constant  Value=2*pi
  Constant1 : Constant  Value=365*24*60*60
  Constant2 : Constant  Value=23.45
  Degrees to Radians : simulink_extras/Transformations/Degrees to Radians
  MatrixMultiply : Product  Multiplication=Matrix(*)
  Mux : Mux  Inputs=3
  Product{,1..3} (4 alike) : Product
  Reciprocal : Product  Inputs=1
  Reshape : Reshape  OutputDimensionality=Column vector (2-D)
  Sin : Trigonometry  Operator=cos
  Sin1 : Trigonometry
  Sin2 : Trigonometry  Operator=cos
  Sin3 : Trigonometry
  S_B : Outport
  S_N : Outport  Port=2
  wires:
  Product3/1 -> Mux/3
  Degrees to Radians/1 -> Sin3/1, Sin2/1
  Constant1/1 -> Reciprocal/1
  Sin2/1 -> Product2/2
  Product/1 -> Product1/1  "n"
  Constant2/1 -> Degrees to Radians/1
  Product1/1 -> Sin/1, Sin1/1  "n*t"
  Product2/1 -> Mux/2
  Sin3/1 -> Product3/2
  Clock/1 -> Product1/2
  Sin1/1 -> Product3/1, Product2/1
  Constant/1 -> Product/1
  Sin/1 -> Mux/1
  Reciprocal/1 -> Product/2
  Mux/1 -> Reshape/1
  A_B_N/1 -> MatrixMultiply/1
  MatrixMultiply/1 -> S_B/1
  Reshape/1 -> S_N/1, MatrixMultiply/2

== system uncontrolled_group24/Desturbances/External Torques/Solar radiation/Torque arm MB ==
  note: creo il vettore somma che ha per colonna i raggi vettori che collegano il CM del MB con i centri illuminati delle facce nel caso che il sole sia nelle 4 posizioni.
  MB : Inport
  A_vect : Inport  Port=2
  S_B : Inport  Port=3
  pointer : Inport  Port=4
  Demux : Demux  Outputs=3
  Reshape : Reshape  OutputDimensionality=Customize  OutputDimensions=[3,3]
  Transpose : Math  Operator=transpose
  Vector Concatenate : Concatenate  NumInputs=3
  creazione raggi vettore tra CM MB e centro facce illuminate della faccia che ha come normale l'asse i : Subsystem
  creazione raggi vettore tra CM MB e centro facce illuminate della faccia che ha come normale l'asse j : Subsystem
  creazione raggi vettore tra CM MB e centro facce illuminate della faccia che ha come normale l'asse k : Subsystem
  dist : Outport
  wires:
  pointer/1 -> Demux/1
  [x] -> creazione raggi vettore tra CM MB e centro facce illuminate della faccia che ha come normale l'asse i/4(pointer)
  [A_vect] -> creazione raggi vettore tra CM MB e centro facce illuminate della faccia che ha come normale l'asse i/3(A_vect)
  [MB] -> creazione raggi vettore tra CM MB e centro facce illuminate della faccia che ha come normale l'asse k/2(MB)
  [y] -> creazione raggi vettore tra CM MB e centro facce illuminate della faccia che ha come normale l'asse j/4(pointer)
  S_B/1 -> [S_B]
  [A_vect] -> creazione raggi vettore tra CM MB e centro facce illuminate della faccia che ha come normale l'asse k/3(A_vect)
  [MB] -> creazione raggi vettore tra CM MB e centro facce illuminate della faccia che ha come normale l'asse j/2(MB)
  A_vect/1 -> [A_vect]
  MB/1 -> [MB]
  [MB] -> creazione raggi vettore tra CM MB e centro facce illuminate della faccia che ha come normale l'asse i/2(MB)
  Reshape/1 -> Transpose/1
  Transpose/1 -> dist/1
  [S_B] -> creazione raggi vettore tra CM MB e centro facce illuminate della faccia che ha come normale l'asse k/1(S_B)
  Demux/1 -> [x]
  Demux/3 -> [z]
  [S_B] -> creazione raggi vettore tra CM MB e centro facce illuminate della faccia che ha come normale l'asse j/1(S_B)
  [z] -> creazione raggi vettore tra CM MB e centro facce illuminate della faccia che ha come normale l'asse k/4(pointer)
  Vector Concatenate/1 -> Reshape/1  "vectors x, y, z"
  [A_vect] -> creazione raggi vettore tra CM MB e centro facce illuminate della faccia che ha come normale l'asse j/3(A_vect)
  [S_B] -> creazione raggi vettore tra CM MB e centro facce illuminate della faccia che ha come normale l'asse i/1(S_B)
  Demux/2 -> [y]
  creazione raggi vettore tra CM MB e centro facce illuminate della faccia che ha come normale l'asse k/1(Out1) -> Vector Concatenate/3
  creazione raggi vettore tra CM MB e centro facce illuminate della faccia che ha come normale l'asse j/1(Out1) -> Vector Concatenate/2
  creazione raggi vettore tra CM MB e centro facce illuminate della faccia che ha come normale l'asse i/1(Out1) -> Vector Concatenate/1

== system uncontrolled_group24/Desturbances/External Torques/Solar radiation/Torque arm SP ==
  SP : Inport
  A_vect_SP : Inport  Port=2
  S_B : Inport  Port=3
  pointer_SP : Inport  Port=4
  r_SP1 : Inport  Port=5
  r_SP2 : Inport  Port=6
  Add : Sum
  Add1 : Sum
  Reshape : Reshape  OutputDimensionality=Customize  OutputDimensions=[2,3]
  Vector Concatenate : Concatenate
  creazione raggi vettore tra CM SP e centro facce illuminate della faccia che ha come normale l'asse j : Subsystem
  distance : Outport
  wires:
  Reshape/1 -> distance/1
  SP/1 -> [SP]
  A_vect_SP/1 -> [A_vect_SP]
  S_B/1 -> [S_B]
  pointer_SP/1 -> [pointer_SP]
  r_SP1/1 -> [r_SP1]
  r_SP2/1 -> [r_SP2]
  [S_B] -> creazione raggi vettore tra CM SP e centro facce illuminate della faccia che ha come normale l'asse j/1(S_B)
  [SP] -> creazione raggi vettore tra CM SP e centro facce illuminate della faccia che ha come normale l'asse j/2(SP)
  [A_vect_SP] -> creazione raggi vettore tra CM SP e centro facce illuminate della faccia che ha come normale l'asse j/3(A_vect)
  [pointer_SP] -> creazione raggi vettore tra CM SP e centro facce illuminate della faccia che ha come normale l'asse j/4(pointer)
  creazione raggi vettore tra CM SP e centro facce illuminate della faccia che ha come normale l'asse j/1(distance) -> [distance]
  Vector Concatenate/1 -> Reshape/1
  Add/1 -> Vector Concatenate/1
  [distance] -> Add/1
  [r_SP1] -> Add/2
  [r_SP2] -> Add1/2
  [distance] -> Add1/1
  Add1/1 -> Vector Concatenate/2

== system uncontrolled_group24/Desturbances/External Torques/SRP con frecce/SRP/Subsystem ==
  r_s_B : Inport
  Add22 : Sum
  Add23 : Sum
  Add24 : Sum  Inputs=+-
  Constant30 : Constant  Value=s2.A
  Constant31 : Constant  Value=s2.n
  Constant44 : Constant  Value=rho_d_body
  Constant47 : Constant  Value=s2.n
  Constant50 : Constant
  Constant51 : Constant  Value=rho_s_body
  Constant52 : Constant  Value=s2.r
  Cross Product10 : vrlib/Utilities/Cross Product
  Dot Product10 : DotProduct  OutDataTypeStr=Inherit: Inherit via internal rule
  Gain40 : Gain  Gain=0
  Gain41 : Gain  Gain=-P
  Gain42 : Gain  Gain=2
  Gain43 : Gain  Gain=rho_s_body
  Product{1..4} (4 alike) : Product
  Switch10 : Switch  Criteria=u2 > Threshold  SaturateOnIntegerOverflow=off  InputSameDT=off
  pan2 : Outport
  wires:
  Constant50/1 -> Add24/1
  Gain42/1 -> Gain43/1
  Cross Product10/1 -> pan2/1
  Gain43/1 -> Add22/2
  Constant52/1 -> Cross Product10/1
  Add22/1 -> Product2/2
  Gain41/1 -> Product1/2
  Gain40/1 -> Switch10/3
  Dot Product10/1 -> Gain40/1, Switch10/1, Switch10/2
  Product2/1 -> Add23/2
  Constant31/1 -> Dot Product10/2
  Constant51/1 -> Add24/2
  Add24/1 -> Product3/2
  Product3/1 -> Add23/1
  Constant44/1 -> Add22/1
  r_s_B/1 -> Product3/1, Dot Product10/1
  Product1/1 -> Product4/1
  Constant47/1 -> Product2/1
  Switch10/1 -> Gain41/1, Gain42/1
  Constant30/1 -> Product1/1
  Product4/1 -> Cross Product10/2
  Add23/1 -> Product4/2

== system uncontrolled_group24/Desturbances/External Torques/SRP con frecce/SRP/Subsystem1 ==
  r_s_B : Inport
  Add22 : Sum
  Add23 : Sum
  Add24 : Sum  Inputs=+-
  Constant30 : Constant  Value=s3.A
  Constant31 : Constant  Value=s3.n
  Constant44 : Constant  Value=rho_d_body
  Constant47 : Constant  Value=s3.n
  Constant50 : Constant
  Constant51 : Constant  Value=rho_s_body
  Constant52 : Constant  Value=s3.r
  Cross Product10 : vrlib/Utilities/Cross Product
  Dot Product10 : DotProduct  OutDataTypeStr=Inherit: Inherit via internal rule
  Gain40 : Gain  Gain=0
  Gain41 : Gain  Gain=-P
  Gain42 : Gain  Gain=2
  Gain43 : Gain  Gain=rho_s_body
  Product{1..4} (4 alike) : Product
  Switch10 : Switch  Criteria=u2 > Threshold  SaturateOnIntegerOverflow=off  InputSameDT=off
  pan3 : Outport
  wires:
  Add23/1 -> Product4/2
  Product4/1 -> Cross Product10/2
  Constant30/1 -> Product1/1
  Switch10/1 -> Gain42/1, Gain41/1
  Constant47/1 -> Product2/1
  Product1/1 -> Product4/1
  r_s_B/1 -> Dot Product10/1, Product3/1
  Constant44/1 -> Add22/1
  Product3/1 -> Add23/1
  Add24/1 -> Product3/2
  Constant51/1 -> Add24/2
  Constant31/1 -> Dot Product10/2
  Product2/1 -> Add23/2
  Dot Product10/1 -> Switch10/2, Switch10/1, Gain40/1
  Gain40/1 -> Switch10/3
  Gain41/1 -> Product1/2
  Add22/1 -> Product2/2
  Constant52/1 -> Cross Product10/1
  Gain43/1 -> Add22/2
  Cross Product10/1 -> pan3/1
  Gain42/1 -> Gain43/1
  Constant50/1 -> Add24/1

== system uncontrolled_group24/Desturbances/External Torques/SRP con frecce/SRP/Subsystem2 ==
  r_s_B : Inport
  Add22 : Sum
  Add23 : Sum
  Add24 : Sum  Inputs=+-
  Constant30 : Constant  Value=s1.A
  Constant31 : Constant  Value=s1.n
  Constant44 : Constant  Value=rho_d_body
  Constant47 : Constant  Value=s1.n
  Constant50 : Constant
  Constant51 : Constant  Value=rho_s_body
  Constant52 : Constant  Value=s1.r
  Cross Product10 : vrlib/Utilities/Cross Product
  Dot Product10 : DotProduct  OutDataTypeStr=Inherit: Inherit via internal rule
  Gain40 : Gain  Gain=0
  Gain41 : Gain  Gain=-P
  Gain42 : Gain  Gain=2
  Gain43 : Gain  Gain=rho_s_body
  Product{1..4} (4 alike) : Product
  Switch10 : Switch  Criteria=u2 > Threshold  SaturateOnIntegerOverflow=off  InputSameDT=off
  pan1 : Outport
  wires:
  Add23/1 -> Product4/2
  Product4/1 -> Cross Product10/2
  Constant30/1 -> Product1/1
  Switch10/1 -> Gain42/1, Gain41/1
  Constant47/1 -> Product2/1
  Product1/1 -> Product4/1
  r_s_B/1 -> Dot Product10/1, Product3/1
  Constant44/1 -> Add22/1
  Product3/1 -> Add23/1
  Add24/1 -> Product3/2
  Constant51/1 -> Add24/2
  Constant31/1 -> Dot Product10/2
  Product2/1 -> Add23/2
  Dot Product10/1 -> Switch10/2, Switch10/1, Gain40/1
  Gain40/1 -> Switch10/3
  Gain41/1 -> Product1/2
  Add22/1 -> Product2/2
  Constant52/1 -> Cross Product10/1
  Gain43/1 -> Add22/2
  Cross Product10/1 -> pan1/1
  Gain42/1 -> Gain43/1
  Constant50/1 -> Add24/1

== system uncontrolled_group24/Desturbances/External Torques/SRP con frecce/SRP/Subsystem3 ==
  r_s_B : Inport
  Add22 : Sum
  Add23 : Sum
  Add24 : Sum  Inputs=+-
  Constant30 : Constant  Value=s5.A
  Constant31 : Constant  Value=s5.n
  Constant44 : Constant  Value=rho_d_body
  Constant47 : Constant  Value=s5.n
  Constant50 : Constant
  Constant51 : Constant  Value=rho_s_body
  Constant52 : Constant  Value=s5.r
  Cross Product10 : vrlib/Utilities/Cross Product
  Dot Product10 : DotProduct  OutDataTypeStr=Inherit: Inherit via internal rule
  Gain40 : Gain  Gain=0
  Gain41 : Gain  Gain=-P
  Gain42 : Gain  Gain=2
  Gain43 : Gain  Gain=rho_s_body
  Product{1..4} (4 alike) : Product
  Switch10 : Switch  Criteria=u2 > Threshold  SaturateOnIntegerOverflow=off  InputSameDT=off
  pan5 : Outport
  wires:
  Constant50/1 -> Add24/1
  Gain42/1 -> Gain43/1
  Cross Product10/1 -> pan5/1
  Gain43/1 -> Add22/2
  Constant52/1 -> Cross Product10/1
  Add22/1 -> Product2/2
  Gain41/1 -> Product1/2
  Gain40/1 -> Switch10/3
  Dot Product10/1 -> Gain40/1, Switch10/1, Switch10/2
  Product2/1 -> Add23/2
  Constant31/1 -> Dot Product10/2
  Constant51/1 -> Add24/2
  Add24/1 -> Product3/2
  Product3/1 -> Add23/1
  Constant44/1 -> Add22/1
  r_s_B/1 -> Product3/1, Dot Product10/1
  Product1/1 -> Product4/1
  Constant47/1 -> Product2/1
  Switch10/1 -> Gain41/1, Gain42/1
  Constant30/1 -> Product1/1
  Product4/1 -> Cross Product10/2
  Add23/1 -> Product4/2

== system uncontrolled_group24/Desturbances/External Torques/SRP con frecce/SRP/Subsystem4 ==
  r_s_B : Inport
  Add22 : Sum
  Add23 : Sum
  Add24 : Sum  Inputs=+-
  Constant30 : Constant  Value=s4.A
  Constant31 : Constant  Value=s4.n
  Constant44 : Constant  Value=rho_d_body
  Constant47 : Constant  Value=s4.n
  Constant50 : Constant
  Constant51 : Constant  Value=rho_s_body
  Constant52 : Constant  Value=s4.r
  Cross Product10 : vrlib/Utilities/Cross Product
  Dot Product10 : DotProduct  OutDataTypeStr=Inherit: Inherit via internal rule
  Gain40 : Gain  Gain=0
  Gain41 : Gain  Gain=-P
  Gain42 : Gain  Gain=2
  Gain43 : Gain  Gain=rho_s_body
  Product{1..4} (4 alike) : Product
  Switch10 : Switch  Criteria=u2 > Threshold  SaturateOnIntegerOverflow=off  InputSameDT=off
  pan4 : Outport
  wires:
  Constant50/1 -> Add24/1
  Gain42/1 -> Gain43/1
  Cross Product10/1 -> pan4/1
  Gain43/1 -> Add22/2
  Constant52/1 -> Cross Product10/1
  Add22/1 -> Product2/2
  Gain41/1 -> Product1/2
  Gain40/1 -> Switch10/3
  Dot Product10/1 -> Gain40/1, Switch10/1, Switch10/2
  Product2/1 -> Add23/2
  Constant31/1 -> Dot Product10/2
  Constant51/1 -> Add24/2
  Add24/1 -> Product3/2
  Product3/1 -> Add23/1
  Constant44/1 -> Add22/1
  r_s_B/1 -> Product3/1, Dot Product10/1
  Product1/1 -> Product4/1
  Constant47/1 -> Product2/1
  Switch10/1 -> Gain41/1, Gain42/1
  Constant30/1 -> Product1/1
  Product4/1 -> Cross Product10/2
  Add23/1 -> Product4/2

== system uncontrolled_group24/Desturbances/External Torques/SRP con frecce/SRP/Subsystem5 ==
  r_s_B : Inport
  Add22 : Sum
  Add23 : Sum
  Add24 : Sum  Inputs=+-
  Constant30 : Constant  Value=pan1.A1
  Constant31 : Constant  Value=pan1.n1
  Constant44 : Constant  Value=rho_d_sp
  Constant47 : Constant  Value=pan1.n1
  Constant50 : Constant
  Constant51 : Constant  Value=rho_s_sp
  Constant52 : Constant  Value=pan1.r1
  Cross Product10 : vrlib/Utilities/Cross Product
  Dot Product10 : DotProduct  OutDataTypeStr=Inherit: Inherit via internal rule
  Gain40 : Gain  Gain=0
  Gain41 : Gain  Gain=-P
  Gain42 : Gain  Gain=2
  Gain43 : Gain  Gain=rho_s_sp
  Product{1..4} (4 alike) : Product
  Switch10 : Switch  Criteria=u2 > Threshold  SaturateOnIntegerOverflow=off  InputSameDT=off
  ps1 : Outport
  wires:
  Add23/1 -> Product4/2
  Product4/1 -> Cross Product10/2
  Constant30/1 -> Product1/1
  Switch10/1 -> Gain42/1, Gain41/1
  Constant47/1 -> Product2/1
  Product1/1 -> Product4/1
  r_s_B/1 -> Dot Product10/1, Product3/1
  Constant44/1 -> Add22/1
  Product3/1 -> Add23/1
  Add24/1 -> Product3/2
  Constant51/1 -> Add24/2
  Constant31/1 -> Dot Product10/2
  Product2/1 -> Add23/2
  Dot Product10/1 -> Switch10/2, Switch10/1, Gain40/1
  Gain40/1 -> Switch10/3
  Gain41/1 -> Product1/2
  Add22/1 -> Product2/2
  Constant52/1 -> Cross Product10/1
  Gain43/1 -> Add22/2
  Cross Product10/1 -> ps1/1
  Gain42/1 -> Gain43/1
  Constant50/1 -> Add24/1

== system uncontrolled_group24/Desturbances/External Torques/SRP con frecce/SRP/Subsystem6 ==
  r_s_B : Inport
  Add22 : Sum
  Add23 : Sum
  Add24 : Sum  Inputs=+-
  Constant30 : Constant  Value=pan1.A2
  Constant31 : Constant  Value=pan1.n2
  Constant44 : Constant  Value=rho_d_sp
  Constant47 : Constant  Value=pan1.n2
  Constant50 : Constant
  Constant51 : Constant  Value=rho_s_sp
  Constant52 : Constant  Value=pan1.r2
  Cross Product10 : vrlib/Utilities/Cross Product
  Dot Product10 : DotProduct  OutDataTypeStr=Inherit: Inherit via internal rule
  Gain40 : Gain  Gain=0
  Gain41 : Gain  Gain=-P
  Gain42 : Gain  Gain=2
  Gain43 : Gain  Gain=rho_s_sp
  Product{1..4} (4 alike) : Product
  Switch10 : Switch  Criteria=u2 > Threshold  SaturateOnIntegerOverflow=off  InputSameDT=off
  ps2 : Outport
  wires:
  Constant50/1 -> Add24/1
  Gain42/1 -> Gain43/1
  Cross Product10/1 -> ps2/1
  Gain43/1 -> Add22/2
  Constant52/1 -> Cross Product10/1
  Add22/1 -> Product2/2
  Gain41/1 -> Product1/2
  Gain40/1 -> Switch10/3
  Dot Product10/1 -> Gain40/1, Switch10/1, Switch10/2
  Product2/1 -> Add23/2
  Constant31/1 -> Dot Product10/2
  Constant51/1 -> Add24/2
  Add24/1 -> Product3/2
  Product3/1 -> Add23/1
  Constant44/1 -> Add22/1
  r_s_B/1 -> Product3/1, Dot Product10/1
  Product1/1 -> Product4/1
  Constant47/1 -> Product2/1
  Switch10/1 -> Gain41/1, Gain42/1
  Constant30/1 -> Product1/1
  Product4/1 -> Cross Product10/2
  Add23/1 -> Product4/2

== system uncontrolled_group24/Desturbances/External Torques/SRP con frecce/SRP/Subsystem7 ==
  r_s_B : Inport
  Add22 : Sum
  Add23 : Sum
  Add24 : Sum  Inputs=+-
  Constant30 : Constant  Value=s6.A
  Constant31 : Constant  Value=s6.n
  Constant44 : Constant  Value=rho_d_body
  Constant47 : Constant  Value=s6.n
  Constant50 : Constant
  Constant51 : Constant  Value=rho_s_body
  Constant52 : Constant  Value=s6.r
  Cross Product10 : vrlib/Utilities/Cross Product
  Dot Product10 : DotProduct  OutDataTypeStr=Inherit: Inherit via internal rule
  Gain40 : Gain  Gain=0
  Gain41 : Gain  Gain=-P
  Gain42 : Gain  Gain=2
  Gain43 : Gain  Gain=rho_s_body
  Product{1..4} (4 alike) : Product
  Switch10 : Switch  Criteria=u2 > Threshold  SaturateOnIntegerOverflow=off  InputSameDT=off
  pan6 : Outport
  wires:
  Constant50/1 -> Add24/1
  Gain42/1 -> Gain43/1
  Cross Product10/1 -> pan6/1
  Gain43/1 -> Add22/2
  Constant52/1 -> Cross Product10/1
  Add22/1 -> Product2/2
  Gain41/1 -> Product1/2
  Gain40/1 -> Switch10/3
  Dot Product10/1 -> Gain40/1, Switch10/1, Switch10/2
  Product2/1 -> Add23/2
  Constant31/1 -> Dot Product10/2
  Constant51/1 -> Add24/2
  Add24/1 -> Product3/2
  Product3/1 -> Add23/1
  Constant44/1 -> Add22/1
  r_s_B/1 -> Product3/1, Dot Product10/1
  Product1/1 -> Product4/1
  Constant47/1 -> Product2/1
  Switch10/1 -> Gain41/1, Gain42/1
  Constant30/1 -> Product1/1
  Product4/1 -> Cross Product10/2
  Add23/1 -> Product4/2

== system uncontrolled_group24/Desturbances/External Torques/SRP con frecce/SRP/Subsystem8 ==
  r_s_B : Inport
  Add22 : Sum
  Add23 : Sum
  Add24 : Sum  Inputs=+-
  Constant30 : Constant  Value=pan2.A2
  Constant31 : Constant  Value=pan2.n2
  Constant44 : Constant  Value=rho_d_sp
  Constant47 : Constant  Value=pan2.n2
  Constant50 : Constant
  Constant51 : Constant  Value=rho_s_sp
  Constant52 : Constant  Value=pan2.r2
  Cross Product10 : vrlib/Utilities/Cross Product
  Dot Product10 : DotProduct  OutDataTypeStr=Inherit: Inherit via internal rule
  Gain40 : Gain  Gain=0
  Gain41 : Gain  Gain=-P
  Gain42 : Gain  Gain=2
  Gain43 : Gain  Gain=rho_s_sp
  Product{1..4} (4 alike) : Product
  Switch10 : Switch  Criteria=u2 > Threshold  SaturateOnIntegerOverflow=off  InputSameDT=off
  ps4 : Outport
  wires:
  Add23/1 -> Product4/2
  Product4/1 -> Cross Product10/2
  Constant30/1 -> Product1/1
  Switch10/1 -> Gain42/1, Gain41/1
  Constant47/1 -> Product2/1
  Product1/1 -> Product4/1
  r_s_B/1 -> Dot Product10/1, Product3/1
  Constant44/1 -> Add22/1
  Product3/1 -> Add23/1
  Add24/1 -> Product3/2
  Constant51/1 -> Add24/2
  Constant31/1 -> Dot Product10/2
  Product2/1 -> Add23/2
  Dot Product10/1 -> Switch10/2, Switch10/1, Gain40/1
  Gain40/1 -> Switch10/3
  Gain41/1 -> Product1/2
  Add22/1 -> Product2/2
  Constant52/1 -> Cross Product10/1
  Gain43/1 -> Add22/2
  Cross Product10/1 -> ps4/1
  Gain42/1 -> Gain43/1
  Constant50/1 -> Add24/1
